simulink subsystem "Controllers"  (R2024b)
settings: Solver=VariableStepAuto  StartTime=0.0  StopTime=10.0  RelTol=1e-3
values from neighbouring files (symbols this model uses):
  CarrierFreq = 150    [init_MMC_HVDC_200.m]
  freq_left = 50    [init_MMC_HVDC_200.m]
  freq_right = 50    [init_MMC_HVDC_200.m]
  Ll = 0.04889    [init_MMC_HVDC_200.m]
  nb_cell = numberOfCell    (= 200)    [init_MMC_HVDC_200.m]
  numberOfCell = 200    [init_MMC_HVDC_200.m]
  P_AC = 1000e6    (= 1000000000)    [init_MMC_HVDC_200.m]
  Rl = 0    [init_MMC_HVDC_200.m]
  Tctrl = Ts    (= 3.5e-05)    [init_MMC_HVDC_200.m]
  Ts = 35e-6    (= 3.5e-05)    [init_MMC_HVDC_200.m]
  V_AC_sec = 320e3    (= 320000)    [init_MMC_HVDC_200.m]
undefined symbols (not defined in the file or in its folder): dend, DiscIntNeverNeededParam, numd
libraries: powerlib_extras x12, simulink x10
(part 3 of 4)

== system Controllers/pulsegen_VBC2/VBC/VBC6 ==
  mode : Inport
  g : Inport  Port=2
  Vc : Inport  Port=3
  ichg : Inport  Port=4
  Nref : Inport  Port=5
  Constant : Constant  Value=numberOfCell
  Demux3 : Demux  Outputs=2
  MATLAB Function : MATLAB Function  TreatAsAtomicUnit=on
  Signal Specification : SignalSpecification  Dimensions=2
  Terminator : Terminator
  Unit Delay : UnitDelay  SampleTime=Ts  HasFrameUpgradeWarning=on
  Unit Delay1 : UnitDelay  SampleTime=Ts  HasFrameUpgradeWarning=on
  go : Outport  VectorParamsAs1DForOutWhenUnconnected=off
  wires:
  Signal Specification/1 -> Unit Delay/1
  g/1 -> MATLAB Function/1(gate_in)
  Vc/1 -> MATLAB Function/2(Vc)
  ichg/1 -> MATLAB Function/3(ichg)
  MATLAB Function/1(go) -> go/1, Unit Delay1/1
  MATLAB Function/2(int) -> Signal Specification/1
  Nref/1 -> MATLAB Function/4(Nref)
  mode/1 -> Demux3/1
  Demux3/2 -> MATLAB Function/5(errV)
  Unit Delay/1 -> MATLAB Function/7(inti)
  Unit Delay1/1 -> MATLAB Function/6(g_his)
  Demux3/1 -> Terminator/1
  Constant/1 -> MATLAB Function/8(nbc)

== system Controllers/pulsegen_VBC2/pulse_gen/PWM ==
  carrier : Inport
  Vcell_ref : Inport  Port=2
  pgmode : Inport  Port=3
  Data Type Conversion : DataTypeConversion  OutDataTypeStr=double  SaturateOnIntegerOverflow=off  RndMeth=Floor
  NLC : Subsystem
  Relational Operator : RelationalOperator  Operator=>  OutDataTypeStr=boolean  RndMeth=Simplest  InputSameDT=off
  Terminator : Terminator
  phase_reorder6 : Selector  InputPortWidth=6  IndexOptions=Index vector (dialog)  Indices=reshape(ones(numberOfCell,1)*[1:6],1,[])  OutputSizes=1
  Upper_gate : Outport  VectorParamsAs1DForOutWhenUnconnected=off
  NLCref : Outport  Port=2  VectorParamsAs1DForOutWhenUnconnected=off
  wires:
  pgmode/1 -> Terminator/1
  Data Type Conversion/1 -> Upper_gate/1
  Relational Operator/1 -> Data Type Conversion/1
  NLC/1(Out1) -> NLCref/1
  Vcell_ref/1 -> NLC/1(In1), phase_reorder6/1
  carrier/1 -> Relational Operator/2
  phase_reorder6/1 -> Relational Operator/1

== system Controllers/pulsegen_VBC2/pulse_gen/carrier_gen ==
  Constant : Constant  DisableCoverage=on  Value=period
  Digital Clock : DigitalClock  SampleTime=Ts
  Look-Up Table1 : Lookup_n-D  DisableCoverage=on  NumberOfTableDimensions=1  BreakpointsForDimension1=rep_seq_t - min(rep_seq_t)  BreakpointsForDimension3=[5, 7]  Table=rep_seq_y  InternalRulePriority=Speed  SaturateOnIntegerOverflow=on
  Math Function : Math  DisableCoverage=on  Operator=mod  SignedPower=on
  Output : SignalConversion  OverrideOpt=off
  Sum : Sum  DisableCoverage=on  Inputs=+-+  InputSameDT=on  SaturateOnIntegerOverflow=on  OutDataTypeStr=Inherit: Same as first input
  offset : Constant  DisableCoverage=on  Value=Noffset
  startTime : S-Function  Commented=on  DisableCoverage=on  FunctionName=sfun_tstart  SFunctionDeploymentMode=off  EnableBusSupport=off
  Out1 : Outport  VectorParamsAs1DForOutWhenUnconnected=off
  wires:
  Sum/1 -> Math Function/1
  Output/1 -> Out1/1
  offset/1 -> Sum/3
  Math Function/1 -> Look-Up Table1/1
  Digital Clock/1 -> Sum/1
  startTime/1 -> Sum/2
  Look-Up Table1/1 -> Output/1
  Constant/1 -> Math Function/2

== system Controllers/sorting Tmuxed/demux/Subsystem1 ==
  In1 : Inport
  Enable : EnablePort
  Out1 : Outport  InitialOutput=1  VectorParamsAs1DForOutWhenUnconnected=off
  wires:
  In1/1 -> Out1/1

== system Controllers/sorting Tmuxed/demux/Subsystem2 ==
  In1 : Inport
  Enable : EnablePort
  Out1 : Outport  InitialOutput=1  VectorParamsAs1DForOutWhenUnconnected=off
  wires:
  In1/1 -> Out1/1

== system Controllers/sorting Tmuxed/demux/Subsystem3 ==
  In1 : Inport
  Enable : EnablePort
  Out1 : Outport  InitialOutput=1  VectorParamsAs1DForOutWhenUnconnected=off
  wires:
  In1/1 -> Out1/1

== system Controllers/sorting Tmuxed/demux/Subsystem4 ==
  In1 : Inport
  Enable : EnablePort
  Out1 : Outport  InitialOutput=1  VectorParamsAs1DForOutWhenUnconnected=off
  wires:
  In1/1 -> Out1/1

== system Controllers/sorting Tmuxed/demux/Subsystem5 ==
  In1 : Inport
  Enable : EnablePort
  Out1 : Outport  InitialOutput=1  VectorParamsAs1DForOutWhenUnconnected=off
  wires:
  In1/1 -> Out1/1

== system Controllers/sorting Tmuxed/demux/Subsystem6 ==
  In1 : Inport
  Enable : EnablePort
  Out1 : Outport  InitialOutput=1  VectorParamsAs1DForOutWhenUnconnected=off
  wires:
  In1/1 -> Out1/1

== system Controllers/sorting Tmuxed/demux1/Subsystem1 ==
  In1 : Inport
  Enable : EnablePort
  Out1 : Outport  InitialOutput=1  VectorParamsAs1DForOutWhenUnconnected=off
  wires:
  In1/1 -> Out1/1

== system Controllers/sorting Tmuxed/demux1/Subsystem2 ==
  In1 : Inport
  Enable : EnablePort
  Out1 : Outport  InitialOutput=1  VectorParamsAs1DForOutWhenUnconnected=off
  wires:
  In1/1 -> Out1/1

== system Controllers/sorting Tmuxed/demux1/Subsystem3 ==
  In1 : Inport
  Enable : EnablePort
  Out1 : Outport  InitialOutput=1  VectorParamsAs1DForOutWhenUnconnected=off
  wires:
  In1/1 -> Out1/1

== system Controllers/sorting Tmuxed/demux1/Subsystem4 ==
  In1 : Inport
  Enable : EnablePort
  Out1 : Outport  InitialOutput=1  VectorParamsAs1DForOutWhenUnconnected=off
  wires:
  In1/1 -> Out1/1

== system Controllers/sorting Tmuxed/demux1/Subsystem5 ==
  In1 : Inport
  Enable : EnablePort
  Out1 : Outport  InitialOutput=1  VectorParamsAs1DForOutWhenUnconnected=off
  wires:
  In1/1 -> Out1/1

== system Controllers/sorting Tmuxed/demux1/Subsystem6 ==
  In1 : Inport
  Enable : EnablePort
  Out1 : Outport  InitialOutput=1  VectorParamsAs1DForOutWhenUnconnected=off
  wires:
  In1/1 -> Out1/1

== system Controllers/VSC controller1/Vdc ctrl/Vdc_ctrler1/PI_d2 ==
  note: Pierre Giroux, Gilbert Sybille
      | Power System Simulation Laboratory
      | IREQ, Hydro-Quebc
  note: Discrete PID Controller
  Error : Inport  SampleTime=Ts
  Discrete-Time Integrator : DiscreteIntegrator  InitialCondition=Init  SampleTime=Ts  LimitOutput=on  UpperSaturationLimit=UpperLimit  LowerSaturationLimit=LowerLimit  ICPrevOutput=DiscIntNeverNeededParam  ICPrevScaledInput=DiscIntNeverNeededParam
  Kp4 : Gain  Gain=Kp  SaturateOnIntegerOverflow=on  SampleTime=Ts  OutDataTypeStr=Inherit: Same as input  ParamDataTypeStr=Inherit: Same as input
  Kp5 : Gain  Gain=Ki  SaturateOnIntegerOverflow=on  SampleTime=Ts  OutDataTypeStr=Inherit: Same as input  ParamDataTypeStr=Inherit: Same as input
  Saturation2 : Saturate  UpperLimit=UpperLimit  LowerLimit=LowerLimit  SampleTime=Ts
  Sum6 : Sum  InputSameDT=on  SaturateOnIntegerOverflow=on  SampleTime=Ts  OutDataTypeStr=Inherit: Same as first input
  Zero-Order Hold : ZeroOrderHold  SampleTime=Ts
  Out : Outport  SampleTime=Ts  InitialOutput=0  VectorParamsAs1DForOutWhenUnconnected=off
  wires:
  Error/1 -> Kp4/1, Kp5/1
  Sum6/1 -> Saturation2/1
  Kp5/1 -> Discrete-Time Integrator/1
  Kp4/1 -> Zero-Order Hold/1
  Discrete-Time Integrator/1 -> Sum6/2  "int"
  Saturation2/1 -> Out/1
  Zero-Order Hold/1 -> Sum6/1  "prop"

== system Controllers/VSC controller1/otherctrl/VSCController_ctrl/ver2 ==
  Vac_ref : Inport
  hisi : Inport  Port=2
  Vcap : Inport  Port=3
  mode : Inport  Port=4
  Iarm : Inport  Port=5
  vdcref : Inport  Port=6
  theda : Inport  Port=7
  Lxpu : Inport  Port=8
  Ictrl : Inport  Port=9
  Ts : Inport  Port=10
  CCSC : Subsystem
  Sum9 : Sum  Inputs=2
  Vsmref : Subsystem
  phase_reorder2 : Selector  InputPortWidth=3  IndexOptions=Index vector (dialog)  Indices=[1 1 2 2 3 3 ]  OutputSizes=1
  ref : Outport  OutputWhenDisabled=reset  InitialOutput=0
  hiso : Outport  Port=2  OutputWhenDisabled=reset  InitialOutput=0
  wires:
  Lxpu/1 -> CCSC/6(Lxpu)
  CCSC/2(hiso) -> hiso/1
  Ictrl/1 -> CCSC/5(Ictrl)
  Ts/1 -> CCSC/4(Ts)
  hisi/1 -> CCSC/3(hisi)
  mode/1 -> Vsmref/2(mode)  "0: voltage mode (vdc follow Vcap) 1: balance mode"
  Sum9/1 -> ref/1  "a1a2b1b2c1c2"
  Vac_ref/1 -> Vsmref/1(Vacref)
  Vcap/1 -> Vsmref/3(Vcap)
  Vsmref/1(Vsmref) -> Sum9/1  "a1a2b1b2c1c2"
  vdcref/1 -> Vsmref/4(vdcref)
  phase_reorder2/1 -> Sum9/2
  CCSC/1(error) -> phase_reorder2/1
  theda/1 -> CCSC/1(Theta)
  Iarm/1 -> CCSC/2(Iarm)

== system Controllers/VSC controller1/pqctrl/dq ctlr/Subsystem1 ==
  Vdq2 : Inport
  PQref : Inport  Port=2
  Fcn7 : Fcn  Expr=(u[1] *u[4]+u[2]*u[5])/u[3]
  Fcn8 : Fcn  Expr=(u[2] *u[4]-u[1]*u[5])/u[3]
  Fcn9 : Fcn  Expr=(u[1] ^2+u[2]^2)
  Mux3 : Mux  Inputs=[2 1 2]
  Mux4 : Mux  Inputs=2
  Saturation : Saturate  UpperLimit=inf  LowerLimit=0.01
  Saturation1 : Saturate  UpperLimit=1.5  LowerLimit=-1.5
  Idqref : Outport  VectorParamsAs1DForOutWhenUnconnected=off
  wires:
  Saturation/1 -> Mux3/2
  PQref/1 -> Mux3/3
  Mux4/1 -> Saturation1/1  "Idqref"
  Fcn8/1 -> Mux4/2
  Fcn7/1 -> Mux4/1
  Fcn9/1 -> Saturation/1
  Mux3/1 -> Fcn7/1, Fcn8/1
  Vdq2/1 -> Mux3/1, Fcn9/1
  Saturation1/1 -> Idqref/1

== system Controllers/VSC controller1/pqctrl/dq ctlr/Vdqref ==
  Vdq2 : Inport
  Idqref : Inport  Port=2
  Fcn7 : Fcn  Expr=(u[2] +u[4]*u[5]+u[3]*u[6])
  Fcn8 : Fcn  Expr=(u[1] +u[3]*u[5]-u[4]*u[6])
  Lxpu : Constant  Value=Lxpu
  Mux3 : Mux
  Mux4 : Mux  Inputs=2
  Rxpu : Constant  Value=Rxpu
  Vdqrefss : Outport  VectorParamsAs1DForOutWhenUnconnected=off
  wires:
  Mux4/1 -> Vdqrefss/1
  Idqref/1 -> Mux3/2
  Vdq2/1 -> Mux3/1
  Fcn7/1 -> Mux4/2  "Vqref"
  Fcn8/1 -> Mux4/1  "Vdref"
  Mux3/1 -> Fcn7/1, Fcn8/1
  Rxpu/1 -> Mux3/3
  Lxpu/1 -> Mux3/4

== system Controllers/VSC controller1/pqctrl/dq ctlr/abc_dq ==
  abc : Inport
  theta : Inport  Port=2
  Mux2 : Mux  Inputs=2
  Selector3 : Selector  InputPortWidth=3  IndexOptions=Index vector (dialog)  Indices=[1 2]  OutputSizes=1
  Trigonometric Function2 : Trigonometry
  Trigonometric Function3 : Trigonometry  Operator=cos
  abc/dq1 : powerlib_extras/Measurements/abc_to_dq0 Transformation
  dq : Outport  VectorParamsAs1DForOutWhenUnconnected=off
  wires:
  Trigonometric Function3/1 -> Mux2/2
  Trigonometric Function2/1 -> Mux2/1
  theta/1 -> Trigonometric Function2/1, Trigonometric Function3/1
  Mux2/1 -> abc/dq1/2
  abc/dq1/1 -> Selector3/1
  Selector3/1 -> dq/1
  abc/1 -> abc/dq1/1

== system Controllers/VSC controller1/pqctrl/dq ctlr/abc_dq1 ==
  abc : Inport
  theta : Inport  Port=2
  Mux2 : Mux  Inputs=2
  Selector3 : Selector  InputPortWidth=3  IndexOptions=Index vector (dialog)  Indices=[1 2]  OutputSizes=1
  Trigonometric Function2 : Trigonometry
  Trigonometric Function3 : Trigonometry  Operator=cos
  abc/dq1 : powerlib_extras/Measurements/abc_to_dq0 Transformation
  dq : Outport  VectorParamsAs1DForOutWhenUnconnected=off
  wires:
  abc/1 -> abc/dq1/1
  Selector3/1 -> dq/1
  abc/dq1/1 -> Selector3/1
  Mux2/1 -> abc/dq1/2
  theta/1 -> Trigonometric Function3/1, Trigonometric Function2/1
  Trigonometric Function2/1 -> Mux2/1
  Trigonometric Function3/1 -> Mux2/2

== system Controllers/VSC controller1/pqctrl/dq ctlr/measure ==
  note: this is to validate Rxpu and Lxpu which make PI(error) almost zero,
      | i.e. the delay is properly set
      |
      | or to calculate Rxpu and Lxpu which make PI(error) zero
      | when input are in steady state
      |
      | when change the P,Q ref,
      | the results should be same if delay is properly cancelled
  A=X-V : Inport
  Idqref : Inport  Port=2
  Display1 : Display
      settings: Decimation=200
  Fcn7 : Fcn  Expr=(u[2] *u[3]-u[1]*u[4])/(u[3]^2+u[4]^2)
  Fcn8 : Fcn  Expr=(u[1] *u[3]+u[2]*u[4])/(u[3]^2+u[4]^2)
  Mux3 : Mux  Inputs=2
  Mux4 : Mux  Inputs=2
  wires:
  Mux4/1 -> Display1/1
  Idqref/1 -> Mux3/2
  A=X-V/1 -> Mux3/1
  Fcn7/1 -> Mux4/2  "Lxpu"
  Fcn8/1 -> Mux4/1  "Rxpu"
  Mux3/1 -> Fcn7/1, Fcn8/1

== system Controllers/VSC controller2/Vdc ctrl/Vdc_ctrler1/PI_d2 ==
  note: Discrete PID Controller
  note: Pierre Giroux, Gilbert Sybille
      | Power System Simulation Laboratory
      | IREQ, Hydro-Quebc
  Error : Inport  SampleTime=Ts
  Discrete-Time Integrator : DiscreteIntegrator  InitialCondition=Init  SampleTime=Ts  LimitOutput=on  UpperSaturationLimit=UpperLimit  LowerSaturationLimit=LowerLimit  ICPrevOutput=DiscIntNeverNeededParam  ICPrevScaledInput=DiscIntNeverNeededParam
  Kp4 : Gain  Gain=Kp  SaturateOnIntegerOverflow=on  SampleTime=Ts  OutDataTypeStr=Inherit: Same as input  ParamDataTypeStr=Inherit: Same as input
  Kp5 : Gain  Gain=Ki  SaturateOnIntegerOverflow=on  SampleTime=Ts  OutDataTypeStr=Inherit: Same as input  ParamDataTypeStr=Inherit: Same as input
  Saturation2 : Saturate  UpperLimit=UpperLimit  LowerLimit=LowerLimit  SampleTime=Ts
  Sum6 : Sum  InputSameDT=on  SaturateOnIntegerOverflow=on  SampleTime=Ts  OutDataTypeStr=Inherit: Same as first input
  Zero-Order Hold : ZeroOrderHold  SampleTime=Ts
  Out : Outport  SampleTime=Ts  InitialOutput=0  VectorParamsAs1DForOutWhenUnconnected=off
  wires:
  Zero-Order Hold/1 -> Sum6/1  "prop"
  Saturation2/1 -> Out/1
  Discrete-Time Integrator/1 -> Sum6/2  "int"
  Kp4/1 -> Zero-Order Hold/1
  Kp5/1 -> Discrete-Time Integrator/1
  Sum6/1 -> Saturation2/1
  Error/1 -> Kp5/1, Kp4/1

== system Controllers/VSC controller2/otherctrl/VSCController_ctrl/ver2 ==
  Vac_ref : Inport
  hisi : Inport  Port=2
  Vcap : Inport  Port=3
  mode : Inport  Port=4
  Iarm : Inport  Port=5
  vdcref : Inport  Port=6
  theda : Inport  Port=7
  Lxpu : Inport  Port=8
  Ictrl : Inport  Port=9
  Ts : Inport  Port=10
  CCSC : Subsystem
  Sum9 : Sum  Inputs=2
  Vsmref : Subsystem
  phase_reorder2 : Selector  InputPortWidth=3  IndexOptions=Index vector (dialog)  Indices=[1 1 2 2 3 3 ]  OutputSizes=1
  ref : Outport  OutputWhenDisabled=reset  InitialOutput=0
  hiso : Outport  Port=2  OutputWhenDisabled=reset  InitialOutput=0
  wires:
  Lxpu/1 -> CCSC/6(Lxpu)
  CCSC/2(hiso) -> hiso/1
  Ictrl/1 -> CCSC/5(Ictrl)
  Ts/1 -> CCSC/4(Ts)
  hisi/1 -> CCSC/3(hisi)
  mode/1 -> Vsmref/2(mode)  "0: voltage mode (vdc follow Vcap) 1: balance mode"
  Sum9/1 -> ref/1  "a1a2b1b2c1c2"
  Vac_ref/1 -> Vsmref/1(Vacref)
  Vcap/1 -> Vsmref/3(Vcap)
  Vsmref/1(Vsmref) -> Sum9/1  "a1a2b1b2c1c2"
  vdcref/1 -> Vsmref/4(vdcref)
  phase_reorder2/1 -> Sum9/2
  CCSC/1(error) -> phase_reorder2/1
  theda/1 -> CCSC/1(Theta)
  Iarm/1 -> CCSC/2(Iarm)

== system Controllers/VSC controller2/pqctrl/dq ctlr/Subsystem1 ==
  Vdq2 : Inport
  PQref : Inport  Port=2
  Fcn7 : Fcn  Expr=(u[1] *u[4]+u[2]*u[5])/u[3]
  Fcn8 : Fcn  Expr=(u[2] *u[4]-u[1]*u[5])/u[3]
  Fcn9 : Fcn  Expr=(u[1] ^2+u[2]^2)
  Mux3 : Mux  Inputs=[2 1 2]
  Mux4 : Mux  Inputs=2
  Saturation : Saturate  UpperLimit=inf  LowerLimit=0.01
  Saturation1 : Saturate  UpperLimit=1.5  LowerLimit=-1.5
  Idqref : Outport  VectorParamsAs1DForOutWhenUnconnected=off
  wires:
  Saturation1/1 -> Idqref/1
  Vdq2/1 -> Fcn9/1, Mux3/1
  Mux3/1 -> Fcn8/1, Fcn7/1
  Fcn9/1 -> Saturation/1
  Fcn7/1 -> Mux4/1
  Fcn8/1 -> Mux4/2
  Mux4/1 -> Saturation1/1  "Idqref"
  PQref/1 -> Mux3/3
  Saturation/1 -> Mux3/2

== system Controllers/VSC controller2/pqctrl/dq ctlr/Vdqref ==
  Vdq2 : Inport
  Idqref : Inport  Port=2
  Display : Display
      settings: Decimation=50
  Fcn7 : Fcn  Expr=(u[2] +u[4]*u[5]+u[3]*u[6])
  Fcn8 : Fcn  Expr=(u[1] +u[3]*u[5]-u[4]*u[6])
  Lxpu : Constant  Value=Lxpu
  Mux3 : Mux
  Mux4 : Mux  Inputs=2
  Rxpu : Constant  Value=Rxpu
  Vdqrefss : Outport  VectorParamsAs1DForOutWhenUnconnected=off
  wires:
  Lxpu/1 -> Mux3/4
  Rxpu/1 -> Mux3/3
  Mux3/1 -> Display/1, Fcn7/1, Fcn8/1
  Fcn8/1 -> Mux4/1  "Vdref"
  Fcn7/1 -> Mux4/2  "Vqref"
  Vdq2/1 -> Mux3/1
  Idqref/1 -> Mux3/2
  Mux4/1 -> Vdqrefss/1

== system Controllers/VSC controller2/pqctrl/dq ctlr/abc_dq ==
  abc : Inport
  theta : Inport  Port=2
  Mux2 : Mux  Inputs=2
  Selector3 : Selector  InputPortWidth=3  IndexOptions=Index vector (dialog)  Indices=[1 2]  OutputSizes=1
  Trigonometric Function2 : Trigonometry
  Trigonometric Function3 : Trigonometry  Operator=cos
  abc/dq1 : powerlib_extras/Measurements/abc_to_dq0 Transformation
  dq : Outport  VectorParamsAs1DForOutWhenUnconnected=off
  wires:
  abc/1 -> abc/dq1/1
  Selector3/1 -> dq/1
  abc/dq1/1 -> Selector3/1
  Mux2/1 -> abc/dq1/2
  theta/1 -> Trigonometric Function3/1, Trigonometric Function2/1
  Trigonometric Function2/1 -> Mux2/1
  Trigonometric Function3/1 -> Mux2/2

== system Controllers/VSC controller2/pqctrl/dq ctlr/abc_dq1 ==
  abc : Inport
  theta : Inport  Port=2
  Mux2 : Mux  Inputs=2
  Selector3 : Selector  InputPortWidth=3  IndexOptions=Index vector (dialog)  Indices=[1 2]  OutputSizes=1
  Trigonometric Function2 : Trigonometry
  Trigonometric Function3 : Trigonometry  Operator=cos
  abc/dq1 : powerlib_extras/Measurements/abc_to_dq0 Transformation
  dq : Outport  VectorParamsAs1DForOutWhenUnconnected=off
  wires:
  Trigonometric Function3/1 -> Mux2/2
  Trigonometric Function2/1 -> Mux2/1
  theta/1 -> Trigonometric Function2/1, Trigonometric Function3/1
  Mux2/1 -> abc/dq1/2
  abc/dq1/1 -> Selector3/1
  Selector3/1 -> dq/1
  abc/1 -> abc/dq1/1

== system Controllers/pulsegen_VBC1/pulse_gen/PWM/NLC ==
  In1 : Inport
  Bias : Bias  Bias=1  SaturateOnIntegerOverflow=off
  Gain : Gain  Gain=nb_cell/2/2
  Rounding Function : Rounding  Operator=round
  Out1 : Outport  VectorParamsAs1DForOutWhenUnconnected=off
  wires:
  Bias/1 -> Gain/1
  Gain/1 -> Rounding Function/1
  In1/1 -> Bias/1
  Rounding Function/1 -> Out1/1

== system Controllers/pulsegen_VBC2/pulse_gen/PWM/NLC ==
  In1 : Inport
  Bias : Bias  Bias=1  SaturateOnIntegerOverflow=off
  Gain : Gain  Gain=nb_cell/2/2
  Rounding Function : Rounding  Operator=round
  Out1 : Outport  VectorParamsAs1DForOutWhenUnconnected=off
  wires:
  Rounding Function/1 -> Out1/1
  In1/1 -> Bias/1
  Gain/1 -> Rounding Function/1
  Bias/1 -> Gain/1

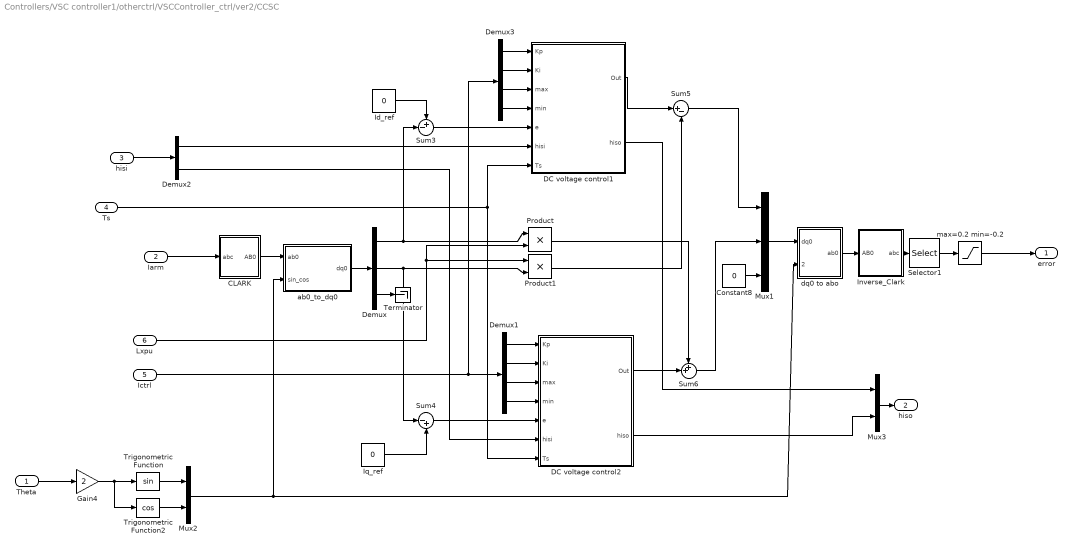
== system Controllers/VSC controller1/otherctrl/VSCController_ctrl/ver2/CCSC ==
  Theta : Inport
  Iarm : Inport  Port=2
  hisi : Inport  Port=3
  Ts : Inport  Port=4
  Ictrl : Inport  Port=5
  Lxpu : Inport  Port=6
  "CLARK  " : Subsystem
  Constant8 : Constant  Value=0
  DC voltage control1 : Subsystem  mask(Integrator  With  External  Dynamic  Limits (Discrete)){}
      mask Display: disp('PI Control')
  DC voltage control2 : Subsystem  mask(Integrator  With  External  Dynamic  Limits (Discrete)){}
      mask Display: disp('PI Control')
  Demux : Demux  Outputs=3
  Demux1 : Demux
  Demux2 : Demux  Outputs=2
  Demux3 : Demux
  Gain4 : Gain  Gain=2
  Id_ref : Constant  Value=0
  Inverse_Clark : Subsystem
  Iq_ref : Constant  Value=0
  Mux1 : Mux  Inputs=3
  Mux2 : Mux  Inputs=2
  Mux3 : Mux  Inputs=2
  Product : Product  RndMeth=Zero
  Product1 : Product  RndMeth=Zero
  Selector1 : Selector  InputPortWidth=3  IndexOptions=Index vector (dialog)  Indices=[1 3 2]  OutputSizes=1
  Sum3 : Sum  Inputs=+-|
  Sum4 : Sum  Inputs=|-+
  Sum5 : Sum  Inputs=|+-
  Sum6 : Sum  Inputs=++|
  Terminator : Terminator
  Trigonometric Function : Trigonometry
  Trigonometric Function2 : Trigonometry  Operator=cos
  ab0_to_dq0 : Subsystem
  dq0 to abo : Subsystem
  max=0.2 min=-0.2 : Saturate  UpperLimit=0.2  LowerLimit=-0.2
  error : Outport
  hiso : Outport  Port=2  InitialOutput=0
  wires:
  Lxpu/1 -> Product1/1, Product/2
  Ts/1 -> DC voltage control2/7(Ts), DC voltage control1/7(Ts)
  Demux2/2 -> DC voltage control2/6(hisi)
  Demux2/1 -> DC voltage control1/6(hisi)
  hisi/1 -> Demux2/1
  DC voltage control2/2(hiso) -> Mux3/2
  DC voltage control1/2(hiso) -> Mux3/1
  Demux1/4 -> DC voltage control2/4(min)
  Demux1/3 -> DC voltage control2/3(max)
  Demux1/2 -> DC voltage control2/2(Ki)
  Demux1/1 -> DC voltage control2/1(Kp)
  Mux3/1 -> hiso/1
  Demux3/4 -> DC voltage control1/4(min)
  Demux3/3 -> DC voltage control1/3(max)
  Demux3/2 -> DC voltage control1/2(Ki)
  Demux3/1 -> DC voltage control1/1(Kp)
  Iarm/1 -> "CLARK  "/1(abc)
  Theta/1 -> Gain4/1
  Gain4/1 -> Trigonometric Function2/1, Trigonometric Function/1
  Trigonometric Function/1 -> Mux2/1
  Trigonometric Function2/1 -> Mux2/2
  Selector1/1 -> max=0.2 min=-0.2/1
  max=0.2 min=-0.2/1 -> error/1
  Inverse_Clark/1(abc) -> Selector1/1
  Constant8/1 -> Mux1/3
  Sum6/1 -> Mux1/2
  Sum5/1 -> Mux1/1
  Mux1/1 -> dq0 to abo/1(dq0)
  dq0 to abo/1(ab0) -> Inverse_Clark/1(AB0)
  DC voltage control2/1(Out) -> Sum6/2
  Product1/1 -> Sum5/2
  DC voltage control1/1(Out) -> Sum5/1
  Product/1 -> Sum6/1
  Sum3/1 -> DC voltage control1/5(e)
  Iq_ref/1 -> Sum4/2
  Id_ref/1 -> Sum3/1
  Demux/2 -> Product1/2, Sum4/1
  Demux/1 -> Product/1, Sum3/2
  Mux2/1 -> dq0 to abo/2(sin_cos), ab0_to_dq0/2(sin_cos)
  ab0_to_dq0/1(dq0) -> Demux/1
  "CLARK  "/1(AB0) -> ab0_to_dq0/1(ab0)
  Sum4/1 -> DC voltage control2/5(e)
  Ictrl/1 -> Demux1/1, Demux3/1
  Demux/3 -> Terminator/1

== system Controllers/VSC controller1/otherctrl/VSCController_ctrl/ver2/Vsmref ==
  Vacref : Inport
  mode : Inport  Port=2
  Vcap : Inport  Port=3
  vdcref : Inport  Port=4
  Constant : Constant
  Divide : Product  Inputs=*/
  Saturation1 : Saturate  UpperLimit=1.25  LowerLimit=0.75
  Subsystem3 : Subsystem
  Switch : Switch  Threshold=0.5  SaturateOnIntegerOverflow=off  InputSameDT=off
  Terminator : Terminator
  Vsmref : Outport
  wires:
  mode/1 -> Switch/2
  Vacref/1 -> Divide/1  "a1b1c1a2b2c2"
  vdcref/1 -> Switch/1
  Vcap/1 -> Switch/3  "a1a2b1b2c1c2"
  Switch/1 -> Saturation1/1  "a1a2b1b2c1c2"
  Divide/1 -> Vsmref/1
  Constant/1 -> Subsystem3/3(Vcap), Subsystem3/2(Vdc), Subsystem3/1(Vacref)
  Saturation1/1 -> Divide/2
  Subsystem3/1(Out1) -> Terminator/1

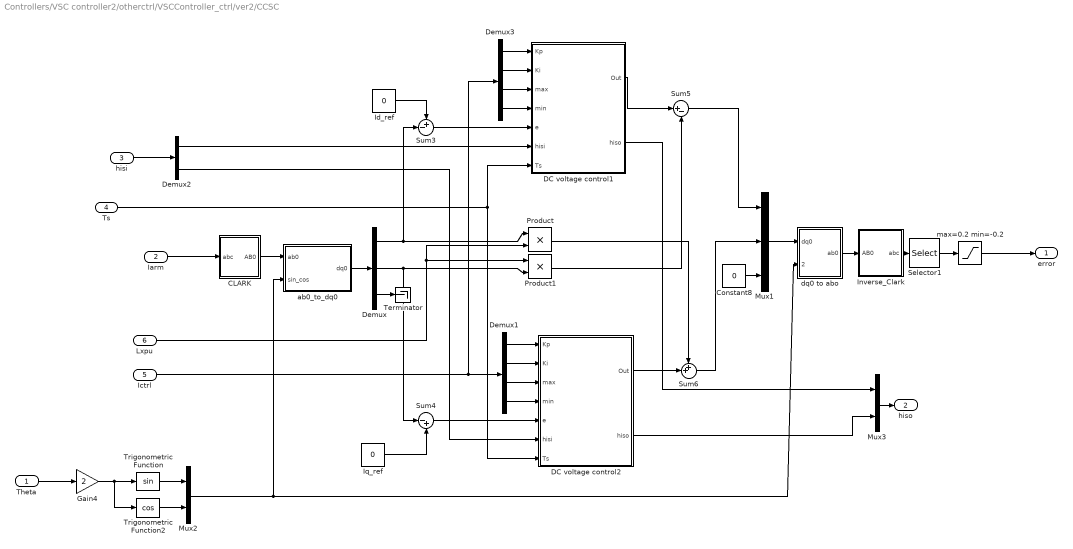
== system Controllers/VSC controller2/otherctrl/VSCController_ctrl/ver2/CCSC ==
  Theta : Inport
  Iarm : Inport  Port=2
  hisi : Inport  Port=3
  Ts : Inport  Port=4
  Ictrl : Inport  Port=5
  Lxpu : Inport  Port=6
  "CLARK  " : Subsystem
  Constant8 : Constant  Value=0
  DC voltage control1 : Subsystem  mask(Integrator  With  External  Dynamic  Limits (Discrete)){}
      mask Display: disp('PI Control')
  DC voltage control2 : Subsystem  mask(Integrator  With  External  Dynamic  Limits (Discrete)){}
      mask Display: disp('PI Control')
  Demux : Demux  Outputs=3
  Demux1 : Demux
  Demux2 : Demux  Outputs=2
  Demux3 : Demux
  Gain4 : Gain  Gain=2
  Id_ref : Constant  Value=0
  Inverse_Clark : Subsystem
  Iq_ref : Constant  Value=0
  Mux1 : Mux  Inputs=3
  Mux2 : Mux  Inputs=2
  Mux3 : Mux  Inputs=2
  Product : Product  RndMeth=Zero
  Product1 : Product  RndMeth=Zero
  Selector1 : Selector  InputPortWidth=3  IndexOptions=Index vector (dialog)  Indices=[1 3 2]  OutputSizes=1
  Sum3 : Sum  Inputs=+-|
  Sum4 : Sum  Inputs=|-+
  Sum5 : Sum  Inputs=|+-
  Sum6 : Sum  Inputs=++|
  Terminator : Terminator
  Trigonometric Function : Trigonometry
  Trigonometric Function2 : Trigonometry  Operator=cos
  ab0_to_dq0 : Subsystem
  dq0 to abo : Subsystem
  max=0.2 min=-0.2 : Saturate  UpperLimit=0.2  LowerLimit=-0.2
  error : Outport
  hiso : Outport  Port=2  InitialOutput=0
  wires:
  Lxpu/1 -> Product1/1, Product/2
  Ts/1 -> DC voltage control2/7(Ts), DC voltage control1/7(Ts)
  Demux2/2 -> DC voltage control2/6(hisi)
  Demux2/1 -> DC voltage control1/6(hisi)
  hisi/1 -> Demux2/1
  DC voltage control2/2(hiso) -> Mux3/2
  DC voltage control1/2(hiso) -> Mux3/1
  Demux1/4 -> DC voltage control2/4(min)
  Demux1/3 -> DC voltage control2/3(max)
  Demux1/2 -> DC voltage control2/2(Ki)
  Demux1/1 -> DC voltage control2/1(Kp)
  Mux3/1 -> hiso/1
  Demux3/4 -> DC voltage control1/4(min)
  Demux3/3 -> DC voltage control1/3(max)
  Demux3/2 -> DC voltage control1/2(Ki)
  Demux3/1 -> DC voltage control1/1(Kp)
  Iarm/1 -> "CLARK  "/1(abc)
  Theta/1 -> Gain4/1
  Gain4/1 -> Trigonometric Function2/1, Trigonometric Function/1
  Trigonometric Function/1 -> Mux2/1
  Trigonometric Function2/1 -> Mux2/2
  Selector1/1 -> max=0.2 min=-0.2/1
  max=0.2 min=-0.2/1 -> error/1
  Inverse_Clark/1(abc) -> Selector1/1
  Constant8/1 -> Mux1/3
  Sum6/1 -> Mux1/2
  Sum5/1 -> Mux1/1
  Mux1/1 -> dq0 to abo/1(dq0)
  dq0 to abo/1(ab0) -> Inverse_Clark/1(AB0)
  DC voltage control2/1(Out) -> Sum6/2
  Product1/1 -> Sum5/2
  DC voltage control1/1(Out) -> Sum5/1
  Product/1 -> Sum6/1
  Sum3/1 -> DC voltage control1/5(e)
  Iq_ref/1 -> Sum4/2
  Id_ref/1 -> Sum3/1
  Demux/2 -> Product1/2, Sum4/1
  Demux/1 -> Product/1, Sum3/2
  Mux2/1 -> dq0 to abo/2(sin_cos), ab0_to_dq0/2(sin_cos)
  ab0_to_dq0/1(dq0) -> Demux/1
  "CLARK  "/1(AB0) -> ab0_to_dq0/1(ab0)
  Sum4/1 -> DC voltage control2/5(e)
  Ictrl/1 -> Demux1/1, Demux3/1
  Demux/3 -> Terminator/1

== system Controllers/VSC controller2/otherctrl/VSCController_ctrl/ver2/Vsmref ==
  Vacref : Inport
  mode : Inport  Port=2
  Vcap : Inport  Port=3
  vdcref : Inport  Port=4
  Constant : Constant
  Divide : Product  Inputs=*/
  Saturation1 : Saturate  UpperLimit=1.25  LowerLimit=0.75
  Subsystem3 : Subsystem
  Switch : Switch  Threshold=0.5  SaturateOnIntegerOverflow=off  InputSameDT=off
  Terminator : Terminator
  Vsmref : Outport
  wires:
  mode/1 -> Switch/2
  Vacref/1 -> Divide/1  "a1b1c1a2b2c2"
  vdcref/1 -> Switch/1
  Vcap/1 -> Switch/3  "a1a2b1b2c1c2"
  Switch/1 -> Saturation1/1  "a1a2b1b2c1c2"
  Divide/1 -> Vsmref/1
  Constant/1 -> Subsystem3/3(Vcap), Subsystem3/2(Vdc), Subsystem3/1(Vacref)
  Saturation1/1 -> Divide/2
  Subsystem3/1(Out1) -> Terminator/1

== system Controllers/VSC controller1/otherctrl/VSCController_ctrl/ver2/CCSC/CLARK   ==
  note: CLARK transformation
  abc : Inport
  Fcn1 : Fcn  Expr=1/sqrt(3)*(u[2] - u[3])
  Fcn2 : Fcn  Expr=1/3*(2*u[1] - u[2] - u[3])
  Fcn3 : Fcn  Expr=1/3*(u[1] + u[2] + u[3])
  Mux : Mux  Inputs=3
  AB0 : Outport
  wires:
  Mux/1 -> AB0/1
  Fcn3/1 -> Mux/3
  Fcn1/1 -> Mux/2
  abc/1 -> Fcn2/1, Fcn3/1, Fcn1/1
  Fcn2/1 -> Mux/1

== system Controllers/VSC controller1/otherctrl/VSCController_ctrl/ver2/CCSC/DC voltage control1 ==
  Kp : Inport
  Ki : Inport  Port=2
  max : Inport  Port=3
  min : Inport  Port=4
  e : Inport  Port=5
  hisi : Inport  Port=6
  Ts : Inport  Port=7
  Demux : Demux  Outputs=[1 2]
  INT : Subsystem
  Mux2 : Mux  Inputs=2
  Product : Product  RndMeth=Zero
  Product1 : Product  RndMeth=Zero
  S6 : Subsystem  mask(Limiter with External Limits){}
      mask Display: disp('      Limiter\n')
  Sum1 : Sum  SaturateOnIntegerOverflow=on
  Sum2 : Sum  Inputs=|+-  SaturateOnIntegerOverflow=on
  Sum3 : Sum  SaturateOnIntegerOverflow=on
  Out : Outport
  hiso : Outport  Port=2  InitialOutput=0
  wires:
  Ts/1 -> INT/3(Ts)
  Demux/2 -> INT/2(hisi)
  Demux/1 -> Sum1/2
  hisi/1 -> Demux/1
  Sum2/1 -> Mux2/1
  INT/2(hiso) -> Mux2/2
  Mux2/1 -> hiso/1
  Ki/1 -> Product/1
  Kp/1 -> Product1/1
  Product1/1 -> Sum3/1
  Product/1 -> Sum3/2
  INT/1(Out) -> Product/2
  Sum3/1 -> Sum2/2, S6/2(In)
  e/1 -> Product1/2, Sum1/1
  Sum1/1 -> INT/1(In)
  max/1 -> S6/1(MAX)
  min/1 -> S6/3(MIN)
  S6/1("  ") -> Out/1, Sum2/1

== system Controllers/VSC controller1/otherctrl/VSCController_ctrl/ver2/CCSC/DC voltage control2 ==
  Kp : Inport
  Ki : Inport  Port=2
  max : Inport  Port=3
  min : Inport  Port=4
  e : Inport  Port=5
  hisi : Inport  Port=6
  Ts : Inport  Port=7
  Demux : Demux  Outputs=[1 2]
  INT : Subsystem
  Mux2 : Mux  Inputs=2
  Product : Product  RndMeth=Zero
  Product1 : Product  RndMeth=Zero
  S6 : Subsystem  mask(Limiter with External Limits){}
      mask Display: disp('      Limiter\n')
  Sum1 : Sum  SaturateOnIntegerOverflow=on
  Sum2 : Sum  Inputs=|+-  SaturateOnIntegerOverflow=on
  Sum3 : Sum  SaturateOnIntegerOverflow=on
  Out : Outport
  hiso : Outport  Port=2  InitialOutput=0
  wires:
  S6/1("  ") -> Sum2/1, Out/1
  min/1 -> S6/3(MIN)
  max/1 -> S6/1(MAX)
  Sum1/1 -> INT/1(In)
  e/1 -> Sum1/1, Product1/2
  Sum3/1 -> S6/2(In), Sum2/2
  INT/1(Out) -> Product/2
  Product/1 -> Sum3/2
  Product1/1 -> Sum3/1
  Kp/1 -> Product1/1
  Ki/1 -> Product/1
  Mux2/1 -> hiso/1
  INT/2(hiso) -> Mux2/2
  Sum2/1 -> Mux2/1
  hisi/1 -> Demux/1
  Demux/1 -> Sum1/2
  Demux/2 -> INT/2(hisi)
  Ts/1 -> INT/3(Ts)

== system Controllers/VSC controller1/otherctrl/VSCController_ctrl/ver2/CCSC/Inverse_Clark ==
  note: Inverse CLARK transformation
  AB0 : Inport
  Fcn1 : Fcn  Expr="1/2*(-u[1]  + sqrt(3)*u[2] + 2*u[3])"
  Fcn2 : Fcn  Expr=(u[1] - u[3])
  Fcn3 : Fcn  Expr=1/2*(-u[1] - sqrt(3)*u[2] + 2*u[3])
  Mux : Mux  Inputs=3
  abc : Outport
  wires:
  Fcn2/1 -> Mux/1
  AB0/1 -> Fcn1/1, Fcn3/1, Fcn2/1
  Fcn1/1 -> Mux/2
  Fcn3/1 -> Mux/3
  Mux/1 -> abc/1

== system Controllers/VSC controller1/otherctrl/VSCController_ctrl/ver2/CCSC/ab0_to_dq0 ==
  note: X0 = X0
  note: Alpha-Beta-zero to dq0
  note: Xd = Xa*sin(wt) - Xb*cos(wt)
  note: Xq = Xa*cos(wt) + Xb*sin(wt)
  ab0 : Inport
  sin_cos : Inport  Port=2
  Demux : Demux  Outputs=2
  Demux1 : Demux  Outputs=3
  Gain3 : Gain  Gain=-1  SaturateOnIntegerOverflow=on  OutDataTypeStr=Inherit: Same as input  ParamDataTypeStr=Inherit: Same as input
  Mux : Mux  Inputs=3
  Product{,1..3} (4 alike) : Product  InputSameDT=on  SaturateOnIntegerOverflow=on  OutDataTypeStr=Inherit: Same as first input
  Sum1 : Sum  Inputs=2  InputSameDT=on  SaturateOnIntegerOverflow=on  OutDataTypeStr=Inherit: Same as first input
  Sum4 : Sum  Inputs=2  InputSameDT=on  SaturateOnIntegerOverflow=on  OutDataTypeStr=Inherit: Same as first input
  dq0 : Outport
  wires:
  Demux1/3 -> Mux/3
  ab0/1 -> Demux1/1
  Mux/1 -> dq0/1
  Product3/1 -> Sum1/2
  Product2/1 -> Sum1/1
  Product1/1 -> Sum4/1
  Demux1/2 -> Product3/1, Product1/1
  Demux/1 -> Product1/2, Product2/2
  Product/1 -> Sum4/2
  Demux1/1 -> Product2/1, Product/1
  Demux/2 -> Product/2, Gain3/1
  sin_cos/1 -> Demux/1
  Sum1/1 -> Mux/1
  Gain3/1 -> Product3/2
  Sum4/1 -> Mux/2

== system Controllers/VSC controller1/otherctrl/VSCController_ctrl/ver2/CCSC/dq0 to abo ==
  note: X0 = X0
  note: dq0 to ab0
  note: Xa = Xd*sin(wt) + Xq*cos(wt)
  note: Xb = -Xd*cos(wt) + Xq*sin(wt)
  dq0 : Inport
  sin_cos : Inport  Port=2
  Demux : Demux  Outputs=2
  Demux1 : Demux  Outputs=3
  Mux : Mux  Inputs=3
  Product{,1..3} (4 alike) : Product  InputSameDT=on  SaturateOnIntegerOverflow=on  OutDataTypeStr=Inherit: Same as first input
  Sum1 : Sum  Inputs=+-  InputSameDT=on  SaturateOnIntegerOverflow=on  OutDataTypeStr=Inherit: Same as first input
  Sum4 : Sum  Inputs=2  InputSameDT=on  SaturateOnIntegerOverflow=on  OutDataTypeStr=Inherit: Same as first input
  ab0 : Outport
  wires:
  dq0/1 -> Demux1/1
  Mux/1 -> ab0/1
  Product3/1 -> Sum1/2
  Product2/1 -> Sum1/1
  Product1/1 -> Sum4/1
  Product/1 -> Sum4/2
  sin_cos/1 -> Demux/1
  Sum4/1 -> Mux/1
  Demux1/1 -> Product1/1, Product3/1
  Demux/1 -> Product1/2, Product2/2
  Demux/2 -> Product/2, Product3/2
  Demux1/2 -> Product/1, Product2/1
  Sum1/1 -> Mux/2
  Demux1/3 -> Mux/3

== system Controllers/VSC controller1/otherctrl/VSCController_ctrl/ver2/Vsmref/Subsystem3 ==
  Vacref : Inport
  Vdc : Inport  Port=2
  Vcap : Inport  Port=3
  Add : Sum
  Bias : Bias  Bias=-1  SaturateOnIntegerOverflow=off
  Divide : Product  Inputs=*/
  Out1 : Outport
  wires:
  Divide/1 -> Bias/1
  Add/1 -> Divide/1
  Vcap/1 -> Divide/2
  Vacref/1 -> Add/1
  Bias/1 -> Out1/1
  Vdc/1 -> Add/2

== system Controllers/VSC controller2/otherctrl/VSCController_ctrl/ver2/CCSC/CLARK   ==
  note: CLARK transformation
  abc : Inport
  Fcn1 : Fcn  Expr=1/sqrt(3)*(u[2] - u[3])
  Fcn2 : Fcn  Expr=1/3*(2*u[1] - u[2] - u[3])
  Fcn3 : Fcn  Expr=1/3*(u[1] + u[2] + u[3])
  Mux : Mux  Inputs=3
  AB0 : Outport
  wires:
  Mux/1 -> AB0/1
  Fcn3/1 -> Mux/3
  Fcn1/1 -> Mux/2
  abc/1 -> Fcn2/1, Fcn3/1, Fcn1/1
  Fcn2/1 -> Mux/1

== system Controllers/VSC controller2/otherctrl/VSCController_ctrl/ver2/CCSC/DC voltage control1 ==
  Kp : Inport
  Ki : Inport  Port=2
  max : Inport  Port=3
  min : Inport  Port=4
  e : Inport  Port=5
  hisi : Inport  Port=6
  Ts : Inport  Port=7
  Demux : Demux  Outputs=[1 2]
  INT : Subsystem
  Mux2 : Mux  Inputs=2
  Product : Product  RndMeth=Zero
  Product1 : Product  RndMeth=Zero
  S6 : Subsystem  mask(Limiter with External Limits){}
      mask Display: disp('      Limiter\n')
  Sum1 : Sum  SaturateOnIntegerOverflow=on
  Sum2 : Sum  Inputs=|+-  SaturateOnIntegerOverflow=on
  Sum3 : Sum  SaturateOnIntegerOverflow=on
  Out : Outport
  hiso : Outport  Port=2  InitialOutput=0
  wires:
  Ts/1 -> INT/3(Ts)
  Demux/2 -> INT/2(hisi)
  Demux/1 -> Sum1/2
  hisi/1 -> Demux/1
  Sum2/1 -> Mux2/1
  INT/2(hiso) -> Mux2/2
  Mux2/1 -> hiso/1
  Ki/1 -> Product/1
  Kp/1 -> Product1/1
  Product1/1 -> Sum3/1
  Product/1 -> Sum3/2
  INT/1(Out) -> Product/2
  Sum3/1 -> Sum2/2, S6/2(In)
  e/1 -> Product1/2, Sum1/1
  Sum1/1 -> INT/1(In)
  max/1 -> S6/1(MAX)
  min/1 -> S6/3(MIN)
  S6/1("  ") -> Out/1, Sum2/1

== system Controllers/VSC controller2/otherctrl/VSCController_ctrl/ver2/CCSC/DC voltage control2 ==
  Kp : Inport
  Ki : Inport  Port=2
  max : Inport  Port=3
  min : Inport  Port=4
  e : Inport  Port=5
  hisi : Inport  Port=6
  Ts : Inport  Port=7
  Demux : Demux  Outputs=[1 2]
  INT : Subsystem
  Mux2 : Mux  Inputs=2
  Product : Product  RndMeth=Zero
  Product1 : Product  RndMeth=Zero
  S6 : Subsystem  mask(Limiter with External Limits){}
      mask Display: disp('      Limiter\n')
  Sum1 : Sum  SaturateOnIntegerOverflow=on
  Sum2 : Sum  Inputs=|+-  SaturateOnIntegerOverflow=on
  Sum3 : Sum  SaturateOnIntegerOverflow=on
  Out : Outport
  hiso : Outport  Port=2  InitialOutput=0
  wires:
  S6/1("  ") -> Sum2/1, Out/1
  min/1 -> S6/3(MIN)
  max/1 -> S6/1(MAX)
  Sum1/1 -> INT/1(In)
  e/1 -> Sum1/1, Product1/2
  Sum3/1 -> S6/2(In), Sum2/2
  INT/1(Out) -> Product/2
  Product/1 -> Sum3/2
  Product1/1 -> Sum3/1
  Kp/1 -> Product1/1
  Ki/1 -> Product/1
  Mux2/1 -> hiso/1
  INT/2(hiso) -> Mux2/2
  Sum2/1 -> Mux2/1
  hisi/1 -> Demux/1
  Demux/1 -> Sum1/2
  Demux/2 -> INT/2(hisi)
  Ts/1 -> INT/3(Ts)

== system Controllers/VSC controller2/otherctrl/VSCController_ctrl/ver2/CCSC/Inverse_Clark ==
  note: Inverse CLARK transformation
  AB0 : Inport
  Fcn1 : Fcn  Expr="1/2*(-u[1]  + sqrt(3)*u[2] + 2*u[3])"
  Fcn2 : Fcn  Expr=(u[1] - u[3])
  Fcn3 : Fcn  Expr=1/2*(-u[1] - sqrt(3)*u[2] + 2*u[3])
  Mux : Mux  Inputs=3
  abc : Outport
  wires:
  Fcn2/1 -> Mux/1
  AB0/1 -> Fcn1/1, Fcn3/1, Fcn2/1
  Fcn1/1 -> Mux/2
  Fcn3/1 -> Mux/3
  Mux/1 -> abc/1

== system Controllers/VSC controller2/otherctrl/VSCController_ctrl/ver2/CCSC/ab0_to_dq0 ==
  note: X0 = X0
  note: Alpha-Beta-zero to dq0
  note: Xd = Xa*sin(wt) - Xb*cos(wt)
  note: Xq = Xa*cos(wt) + Xb*sin(wt)
  ab0 : Inport
  sin_cos : Inport  Port=2
  Demux : Demux  Outputs=2
  Demux1 : Demux  Outputs=3
  Gain3 : Gain  Gain=-1  SaturateOnIntegerOverflow=on  OutDataTypeStr=Inherit: Same as input  ParamDataTypeStr=Inherit: Same as input
  Mux : Mux  Inputs=3
  Product{,1..3} (4 alike) : Product  InputSameDT=on  SaturateOnIntegerOverflow=on  OutDataTypeStr=Inherit: Same as first input
  Sum1 : Sum  Inputs=2  InputSameDT=on  SaturateOnIntegerOverflow=on  OutDataTypeStr=Inherit: Same as first input
  Sum4 : Sum  Inputs=2  InputSameDT=on  SaturateOnIntegerOverflow=on  OutDataTypeStr=Inherit: Same as first input
  dq0 : Outport
  wires:
  Demux1/3 -> Mux/3
  ab0/1 -> Demux1/1
  Mux/1 -> dq0/1
  Product3/1 -> Sum1/2
  Product2/1 -> Sum1/1
  Product1/1 -> Sum4/1
  Demux1/2 -> Product3/1, Product1/1
  Demux/1 -> Product1/2, Product2/2
  Product/1 -> Sum4/2
  Demux1/1 -> Product2/1, Product/1
  Demux/2 -> Product/2, Gain3/1
  sin_cos/1 -> Demux/1
  Sum1/1 -> Mux/1
  Gain3/1 -> Product3/2
  Sum4/1 -> Mux/2

== system Controllers/VSC controller2/otherctrl/VSCController_ctrl/ver2/CCSC/dq0 to abo ==
  note: X0 = X0
  note: dq0 to ab0
  note: Xa = Xd*sin(wt) + Xq*cos(wt)
  note: Xb = -Xd*cos(wt) + Xq*sin(wt)
  dq0 : Inport
  sin_cos : Inport  Port=2
  Demux : Demux  Outputs=2
  Demux1 : Demux  Outputs=3
  Mux : Mux  Inputs=3
  Product{,1..3} (4 alike) : Product  InputSameDT=on  SaturateOnIntegerOverflow=on  OutDataTypeStr=Inherit: Same as first input
  Sum1 : Sum  Inputs=+-  InputSameDT=on  SaturateOnIntegerOverflow=on  OutDataTypeStr=Inherit: Same as first input
  Sum4 : Sum  Inputs=2  InputSameDT=on  SaturateOnIntegerOverflow=on  OutDataTypeStr=Inherit: Same as first input
  ab0 : Outport
  wires:
  dq0/1 -> Demux1/1
  Mux/1 -> ab0/1
  Product3/1 -> Sum1/2
  Product2/1 -> Sum1/1
  Product1/1 -> Sum4/1
  Product/1 -> Sum4/2
  sin_cos/1 -> Demux/1
  Sum4/1 -> Mux/1
  Demux1/1 -> Product1/1, Product3/1
  Demux/1 -> Product1/2, Product2/2
  Demux/2 -> Product/2, Product3/2
  Demux1/2 -> Product/1, Product2/1
  Sum1/1 -> Mux/2
  Demux1/3 -> Mux/3

== system Controllers/VSC controller2/otherctrl/VSCController_ctrl/ver2/Vsmref/Subsystem3 ==
  Vacref : Inport
  Vdc : Inport  Port=2
  Vcap : Inport  Port=3
  Add : Sum
  Bias : Bias  Bias=-1  SaturateOnIntegerOverflow=off
  Divide : Product  Inputs=*/
  Out1 : Outport
  wires:
  Divide/1 -> Bias/1
  Add/1 -> Divide/1
  Vcap/1 -> Divide/2
  Vacref/1 -> Add/1
  Bias/1 -> Out1/1
  Vdc/1 -> Add/2

== system Controllers/VSC controller1/otherctrl/VSCController_ctrl/ver2/CCSC/DC voltage control1/INT ==
  In : Inport
  hisi : Inport  Port=2
  Ts : Inport  Port=3
  Constant : Constant  Value=10
  Constant1 : Constant  Value=-10
  Constant2 : Constant  Value=0.5
  Demux : Demux  Outputs=2
  Mux2 : Mux  Inputs=2
  Product : Product  Inputs=3  SaturateOnIntegerOverflow=on  OutDataTypeStr=Inherit: Same as first input
  S6 : Subsystem  mask(Limiter with External Limits){}
      mask Display: disp('      Limiter\n')
  Sum1 : Sum  InputSameDT=on  SaturateOnIntegerOverflow=on  OutDataTypeStr=Inherit: Same as first input
  Sum2 : Sum  InputSameDT=on  SaturateOnIntegerOverflow=on  OutDataTypeStr=Inherit: Same as first input
  Out : Outport  InitialOutput=0
  hiso : Outport  Port=2  InitialOutput=0
  wires:
  Mux2/1 -> hiso/1
  hisi/1 -> Demux/1
  Ts/1 -> Product/2
  Demux/2 -> Sum2/2
  Sum2/1 -> S6/2(In)
  Product/1 -> Sum2/1
  S6/1("  ") -> Mux2/2, Out/1  "h2"
  Sum1/1 -> Product/3
  Constant2/1 -> Product/1
  Demux/1 -> Sum1/2
  In/1 -> Mux2/1, Sum1/1  "h1"
  Constant/1 -> S6/1(MAX)
  Constant1/1 -> S6/3(MIN)

== system Controllers/VSC controller1/otherctrl/VSCController_ctrl/ver2/CCSC/DC voltage control1/S6 ==
  note: Limiter
      | with external
      | limits
  MAX : Inport
  In : Inport  Port=2
  MIN : Inport  Port=3
  MinMax : MinMax  Function=max  Inputs=2  InputSameDT=on  SaturateOnIntegerOverflow=on
  MinMax1 : MinMax  Inputs=2  InputSameDT=on  SaturateOnIntegerOverflow=on
  "  " : Outport  InitialOutput=0
  wires:
  In/1 -> MinMax1/2
  MinMax/1 -> "  "/1
  MIN/1 -> MinMax/1
  MAX/1 -> MinMax1/1
  MinMax1/1 -> MinMax/2

== system Controllers/VSC controller1/otherctrl/VSCController_ctrl/ver2/CCSC/DC voltage control2/INT ==
  In : Inport
  hisi : Inport  Port=2
  Ts : Inport  Port=3
  Constant : Constant  Value=10
  Constant1 : Constant  Value=-10
  Constant2 : Constant  Value=0.5
  Demux : Demux  Outputs=2
  Mux2 : Mux  Inputs=2
  Product : Product  Inputs=3  SaturateOnIntegerOverflow=on  OutDataTypeStr=Inherit: Same as first input
  S6 : Subsystem  mask(Limiter with External Limits){}
      mask Display: disp('      Limiter\n')
  Sum1 : Sum  InputSameDT=on  SaturateOnIntegerOverflow=on  OutDataTypeStr=Inherit: Same as first input
  Sum2 : Sum  InputSameDT=on  SaturateOnIntegerOverflow=on  OutDataTypeStr=Inherit: Same as first input
  Out : Outport  InitialOutput=0
  hiso : Outport  Port=2  InitialOutput=0
  wires:
  Constant1/1 -> S6/3(MIN)
  Constant/1 -> S6/1(MAX)
  In/1 -> Sum1/1, Mux2/1  "h1"
  Demux/1 -> Sum1/2
  Constant2/1 -> Product/1
  Sum1/1 -> Product/3
  S6/1("  ") -> Out/1, Mux2/2  "h2"
  Product/1 -> Sum2/1
  Sum2/1 -> S6/2(In)
  Demux/2 -> Sum2/2
  Ts/1 -> Product/2
  hisi/1 -> Demux/1
  Mux2/1 -> hiso/1

== system Controllers/VSC controller1/otherctrl/VSCController_ctrl/ver2/CCSC/DC voltage control2/S6 ==
  note: Limiter
      | with external
      | limits
  MAX : Inport
  In : Inport  Port=2
  MIN : Inport  Port=3
  MinMax : MinMax  Function=max  Inputs=2  InputSameDT=on  SaturateOnIntegerOverflow=on
  MinMax1 : MinMax  Inputs=2  InputSameDT=on  SaturateOnIntegerOverflow=on
  "  " : Outport  InitialOutput=0
  wires:
  MinMax1/1 -> MinMax/2
  MAX/1 -> MinMax1/1
  MIN/1 -> MinMax/1
  MinMax/1 -> "  "/1
  In/1 -> MinMax1/2

== system Controllers/VSC controller2/otherctrl/VSCController_ctrl/ver2/CCSC/DC voltage control1/INT ==
  In : Inport
  hisi : Inport  Port=2
  Ts : Inport  Port=3
  Constant : Constant  Value=10
  Constant1 : Constant  Value=-10
  Constant2 : Constant  Value=0.5
  Demux : Demux  Outputs=2
  Mux2 : Mux  Inputs=2
  Product : Product  Inputs=3  SaturateOnIntegerOverflow=on  OutDataTypeStr=Inherit: Same as first input
  S6 : Subsystem  mask(Limiter with External Limits){}
      mask Display: disp('      Limiter\n')
  Sum1 : Sum  InputSameDT=on  SaturateOnIntegerOverflow=on  OutDataTypeStr=Inherit: Same as first input
  Sum2 : Sum  InputSameDT=on  SaturateOnIntegerOverflow=on  OutDataTypeStr=Inherit: Same as first input
  Out : Outport  InitialOutput=0
  hiso : Outport  Port=2  InitialOutput=0
  wires:
  Mux2/1 -> hiso/1
  hisi/1 -> Demux/1
  Ts/1 -> Product/2
  Demux/2 -> Sum2/2
  Sum2/1 -> S6/2(In)
  Product/1 -> Sum2/1
  S6/1("  ") -> Mux2/2, Out/1  "h2"
  Sum1/1 -> Product/3
  Constant2/1 -> Product/1
  Demux/1 -> Sum1/2
  In/1 -> Mux2/1, Sum1/1  "h1"
  Constant/1 -> S6/1(MAX)
  Constant1/1 -> S6/3(MIN)

== system Controllers/VSC controller2/otherctrl/VSCController_ctrl/ver2/CCSC/DC voltage control1/S6 ==
  note: Limiter
      | with external
      | limits
  MAX : Inport
  In : Inport  Port=2
  MIN : Inport  Port=3
  MinMax : MinMax  Function=max  Inputs=2  InputSameDT=on  SaturateOnIntegerOverflow=on
  MinMax1 : MinMax  Inputs=2  InputSameDT=on  SaturateOnIntegerOverflow=on
  "  " : Outport  InitialOutput=0
  wires:
  In/1 -> MinMax1/2
  MinMax/1 -> "  "/1
  MIN/1 -> MinMax/1
  MAX/1 -> MinMax1/1
  MinMax1/1 -> MinMax/2

== system Controllers/VSC controller2/otherctrl/VSCController_ctrl/ver2/CCSC/DC voltage control2/INT ==
  In : Inport
  hisi : Inport  Port=2
  Ts : Inport  Port=3
  Constant : Constant  Value=10
  Constant1 : Constant  Value=-10
  Constant2 : Constant  Value=0.5
  Demux : Demux  Outputs=2
  Mux2 : Mux  Inputs=2
  Product : Product  Inputs=3  SaturateOnIntegerOverflow=on  OutDataTypeStr=Inherit: Same as first input
  S6 : Subsystem  mask(Limiter with External Limits){}
      mask Display: disp('      Limiter\n')
  Sum1 : Sum  InputSameDT=on  SaturateOnIntegerOverflow=on  OutDataTypeStr=Inherit: Same as first input
  Sum2 : Sum  InputSameDT=on  SaturateOnIntegerOverflow=on  OutDataTypeStr=Inherit: Same as first input
  Out : Outport  InitialOutput=0
  hiso : Outport  Port=2  InitialOutput=0
  wires:
  Constant1/1 -> S6/3(MIN)
  Constant/1 -> S6/1(MAX)
  In/1 -> Sum1/1, Mux2/1  "h1"
  Demux/1 -> Sum1/2
  Constant2/1 -> Product/1
  Sum1/1 -> Product/3
  S6/1("  ") -> Out/1, Mux2/2  "h2"
  Product/1 -> Sum2/1
  Sum2/1 -> S6/2(In)
  Demux/2 -> Sum2/2
  Ts/1 -> Product/2
  hisi/1 -> Demux/1
  Mux2/1 -> hiso/1

== system Controllers/VSC controller2/otherctrl/VSCController_ctrl/ver2/CCSC/DC voltage control2/S6 ==
  note: Limiter
      | with external
      | limits
  MAX : Inport
  In : Inport  Port=2
  MIN : Inport  Port=3
  MinMax : MinMax  Function=max  Inputs=2  InputSameDT=on  SaturateOnIntegerOverflow=on
  MinMax1 : MinMax  Inputs=2  InputSameDT=on  SaturateOnIntegerOverflow=on
  "  " : Outport  InitialOutput=0
  wires:
  MinMax1/1 -> MinMax/2
  MAX/1 -> MinMax1/1
  MIN/1 -> MinMax/1
  MinMax/1 -> "  "/1
  In/1 -> MinMax1/2

== system Controllers/VSC controller1/otherctrl/VSCController_ctrl/ver2/CCSC/DC voltage control1/INT/S6 ==
  note: Limiter
      | with external
      | limits
  MAX : Inport
  In : Inport  Port=2
  MIN : Inport  Port=3
  MinMax : MinMax  Function=max  Inputs=2  InputSameDT=on  SaturateOnIntegerOverflow=on
  MinMax1 : MinMax  Inputs=2  InputSameDT=on  SaturateOnIntegerOverflow=on
  "  " : Outport  InitialOutput=0
  wires:
  In/1 -> MinMax1/2
  MinMax/1 -> "  "/1
  MIN/1 -> MinMax/1
  MAX/1 -> MinMax1/1
  MinMax1/1 -> MinMax/2

== system Controllers/VSC controller1/otherctrl/VSCController_ctrl/ver2/CCSC/DC voltage control2/INT/S6 ==
  note: Limiter
      | with external
      | limits
  MAX : Inport
  In : Inport  Port=2
  MIN : Inport  Port=3
  MinMax : MinMax  Function=max  Inputs=2  InputSameDT=on  SaturateOnIntegerOverflow=on
  MinMax1 : MinMax  Inputs=2  InputSameDT=on  SaturateOnIntegerOverflow=on
  "  " : Outport  InitialOutput=0
  wires:
  MinMax1/1 -> MinMax/2
  MAX/1 -> MinMax1/1
  MIN/1 -> MinMax/1
  MinMax/1 -> "  "/1
  In/1 -> MinMax1/2

== system Controllers/VSC controller2/otherctrl/VSCController_ctrl/ver2/CCSC/DC voltage control1/INT/S6 ==
  note: Limiter
      | with external
      | limits
  MAX : Inport
  In : Inport  Port=2
  MIN : Inport  Port=3
  MinMax : MinMax  Function=max  Inputs=2  InputSameDT=on  SaturateOnIntegerOverflow=on
  MinMax1 : MinMax  Inputs=2  InputSameDT=on  SaturateOnIntegerOverflow=on
  "  " : Outport  InitialOutput=0
  wires:
  In/1 -> MinMax1/2
  MinMax/1 -> "  "/1
  MIN/1 -> MinMax/1
  MAX/1 -> MinMax1/1
  MinMax1/1 -> MinMax/2

== system Controllers/VSC controller2/otherctrl/VSCController_ctrl/ver2/CCSC/DC voltage control2/INT/S6 ==
  note: Limiter
      | with external
      | limits
  MAX : Inport
  In : Inport  Port=2
  MIN : Inport  Port=3
  MinMax : MinMax  Function=max  Inputs=2  InputSameDT=on  SaturateOnIntegerOverflow=on
  MinMax1 : MinMax  Inputs=2  InputSameDT=on  SaturateOnIntegerOverflow=on
  "  " : Outport  InitialOutput=0
  wires:
  MinMax1/1 -> MinMax/2
  MAX/1 -> MinMax1/1
  MIN/1 -> MinMax/1
  MinMax/1 -> "  "/1
  In/1 -> MinMax1/2

== matlab function Controllers/pulsegen_VBC1/VBC/VBC3/MATLAB Function ==
  data: gate_in input; go output; int output; Vc input; ichg input; Nref input; errV input; g_his input; inti input; nbc input
function [go,int]= fcn(gate_in,Vc,ichg,Nref,errV,g_his,inti, nbc)

go =gate_in;

NbON =sum(gate_in );


int =[0 ; 0 ];


if NbON >=nbc
    go =ones(size(gate_in));
elseif NbON <=0
    go =zeros (size (gate_in ));
else
    if(inti (1 )>=1 )&&(inti (1 )<=nbc )
        g_his (inti (1 ))=inti (2 );
    end
    if length(g_his) ~= nbc
        gg =gate_in ;

    else
        gg =g_his ;
    end
    NbON_his =sum (g_his );
    event =NbON -NbON_his ;
    aloop0 =1 ;
    aloop1 =1 ;
    idx_m0 =1 ; idx_m1 =1 ;
    for ii =[1 :nbc ]
        if(event >=0 ) && (gg(ii) < 0.5 )
            if(aloop0 ==1 )
                if event >1
                    gg(ii )=1 ;
                    event =event -1 ;
                else
                    idx_m0 =ii ;
                    aloop0 =0 ;
                end
            else

                if (ichg >0 )==(Vc(ii )<Vc (idx_m0 ))
                    idx_m0 =ii ;
                end
            end
        elseif (event<=0 )&&(gg(ii )>0.5 )
            if(aloop1 ==1 )
                if event <-1
                    gg(ii )=0 ;
                    event =event +1 ;
                else
                    idx_m1 =ii ;
                    aloop1 =0 ;
                end
            else


                if (ichg >0 )~=(Vc (ii )<Vc (idx_m1 ))
                    idx_m1 =ii ;
                end
            end
        else

        end
    end
    if (event >0 )
        gg (idx_m0 )=event ;
        if event <1
            int (1 )=idx_m0 ;
            int (2 )=1 ;
        end
    elseif (event < 0)
        gg (idx_m1 )=1 +event ;
        if event >-1
            int (1 )=idx_m1 ;
            int (2 )=0 ;
        end
    else
        if(ichg >0 )
            Vdel =-Vc(idx_m0 ) + Vc(idx_m1 );
        else
            Vdel =Vc(idx_m0 ) - Vc(idx_m1 );
        end
        if (Vdel /(Vc(idx_m0 ) + Vc(idx_m1 ))>errV )
            gg (idx_m0 )=1 ;
            gg (idx_m1 )=0 ;
        end
    end
    go =gg ;
end
